simulink model "Simulink_FLC"  (R2022b)
settings: Solver=VariableStepAuto  StartTime=0.0  StopTime=10.0  RelTol=1e-3
values from neighbouring files (symbols this model uses):
  sys_tf = tf(sys_ss)    [Assingment_Model_.m]
libraries: fuzblock x1, simulink x1
settings Model: Creator=Reyan  LastModifiedBy=Reyan

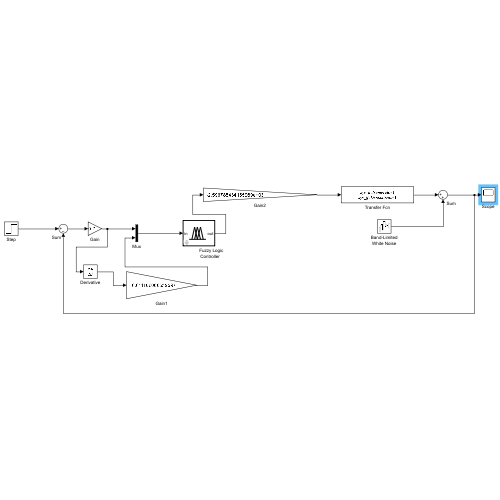
[thumbnail: Simulink's stored preview of the top-level diagram]
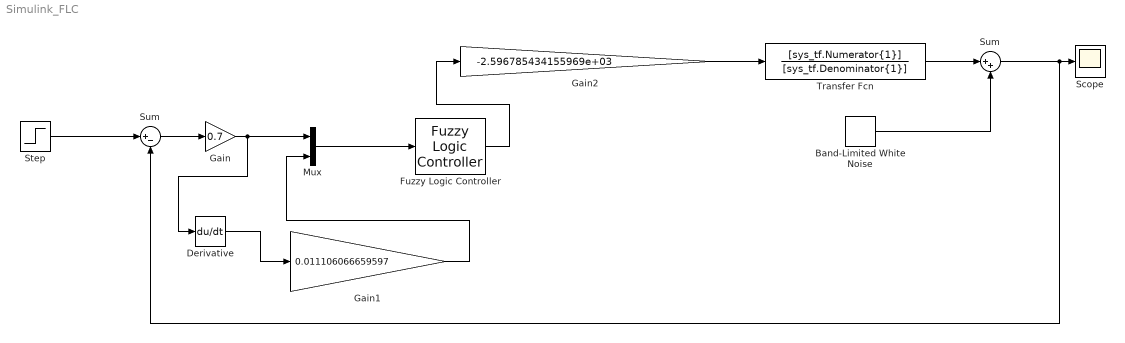
== system Simulink_FLC ==
  "                     Fuzzy Logic Controller" : fuzblock/Fuzzy Logic  Controller  FIS=fis_MLS  OutputSampleNumber=101  DataType=double  FuzzifiedInputs=off  RuleFiringStrengths=off  RuleOutputs=off  AggregatedOutputs=off  SimulateUsing=Interpreted execution  OutOfRangeInputValueMessage=warning  NoRuleFiredMessage=warning  EmptyOutputFuzzySetMessage=warning
  "             Sum" : Sum  Inputs=|++
  Band-Limited White Noise : simulink/Sources/Band-Limited White Noise  Cov=[1e-6]  Ts=0.001  seed=[23341]
  Derivative : Derivative
  Gain : Gain  Gain=0.7
  Gain1 : Gain  Gain=0.011106066659597
  Gain2 : Gain  Gain=-2.596785434155969e+03
  Mux : Mux  Inputs=2
  Scope : Scope
  Step : Step  SampleTime=0
  "Sum           " : Sum  Inputs=|+-
  Transfer Fcn : TransferFcn  Numerator=[sys_tf.Numerator{1}]  Denominator=[sys_tf.Denominator{1}]
  wires:
  Step/1 -> "Sum           "/1
  Mux/1 -> "                     Fuzzy Logic Controller"/1
  "Sum           "/1 -> Gain/1
  Gain/1 -> Derivative/1, Mux/1
  Derivative/1 -> Gain1/1
  Gain1/1 -> Mux/2
  "                     Fuzzy Logic Controller"/1 -> Gain2/1
  Gain2/1 -> Transfer Fcn/1
  Band-Limited White Noise/1 -> "             Sum"/2
  Transfer Fcn/1 -> "             Sum"/1
  "             Sum"/1 -> "Sum           "/2, Scope/1
